simulink model "TENSGwithGFM_electromechanical"  (R2020a)
settings: Solver=VariableStepAuto  StartTime=0.0  StopTime=10.0  FixedStep=0.01  RelTol=1e-3
values from neighbouring files (symbols this model uses):
  GFMInit = GFMSimple_init(resultsac,GFM_in_gidx)    [init.m]
  GSGInit =     [SixGFMconfig.mat]    (also in eightGFMconfig.mat; fourGFMconfig.mat; init.m = SG_init(resultsac,SG_in_gidx); tenGFMconfig.mat)
  Pload = [0 0 0 0 0 0 0 0 0 0 0 0 ... (39 elements, 39x1)]    [SixGFMconfig.mat]    (also in eightGFMconfig.mat; fourGFMconfig.mat; init.m = -resultsac.bus{[CZno,CPno],3}/1000; tenGFMconfig.mat)
  Qload = -resultsac.bus{[CZno,CPno],4}/1000    [init.m]
  Satura = Ses_g(GFM_in_gidx)    [init.m]
  U = [1.0278659059 0.919047677638 0.824047236404 0.914672565668 0.984993620745 0.992890253418 1.00337242347 1.00687710353 1.06162588537 0.973548635627 0.980333735458 0.971076509646 ... (88 elements, 88x1)]    [SixGFMconfig.mat]    (also in eightGFMconfig.mat; fourGFMconfig.mat; init.m = resultsac.bus{:,8}.*exp(1i*(resultsac.bus{:,9})/180*pi); tenGFMconfig.mat)
  Vload = Vbus([CZno,CPno])    [init.m]
  W0 = wB    (= 314.159265359)    [init.m]
  Y_new = [-5.55111512313e-17 -2.77555756156e-17 0 0 0 0 0 0 0 0 0 0 ... (7744 elements, 88x88)]    [SixGFMconfig.mat]    (also in eightGFMconfig.mat; fourGFMconfig.mat; init.m = Y_new([CSno,CPno,GFMother],[CSno,CPno,GFMother]); kron.m = Y)
libraries: eeTransforms x45, simulink_extras x10
(part 3 of 3)

== system TENSGwithGFM_electromechanical/SG1_6 ==
  note: $\[\begin{array}{l} \\ \left\{ \begin{array}{l} {{T'}_d}{{\dot E'}_q} = {E_{fd}} - {{E'}_q} - \left( {{X_d} - {{X'}_d}} \right){I_d}\\ {V_d} = {X_q}{I_q}\\ {V_q} = {{E'}_q} - {{X'}_d}{I_d} \end{array} \right. \end{array}\]$ ${{T'}_d}\dot{{{E'}_q}}=E_{fd}-{E'}_q-(X_d-{X'}_d)I_d \[{V_d} = {X_q}{I_q}\] \[{V_q} = {{E'}_q} - {{X'}_d}{I_d}\]$
  note: AVR
  note: 绕组
  Vxy : Inport
  step : Inport  Port=2
  Clarke to Park Angle Transform1 : eeTransforms/Clarke to Park Angle Transform  AxisAlignment=D-axis
      settings: SourceProductBaseCode=PS
  Constant : Constant  Value=Vref0
  Constant1 : Constant  Value=Pref
  Demux2 : Demux  Outputs=3
  Demux3 : Demux  Outputs=3
  Fcn : Fcn  Expr=sqrt(u(1)^2+u(2)^2)
  Fcn1 : Fcn  Expr=u(1)*u(3)+u(2)*u(4)
  Gain : Gain  Gain=1/Xd1
  Gain1 : Gain  Gain=1/(2*pi)
  Gain10 : Gain  Gain=Xd-Xd1
  Gain12 : Gain  Gain=1/Xq
  Gain13 : Gain  Gain=1/JSG
  Gain14 : Gain  Gain=DSG
  Gain15 : Gain  Gain=W0
  I1 : Constant  Value=0
  I3 : Constant  Value=0
  Integrator1 : Integrator  InitialCondition=theta0
  Integrator5 : Integrator
  Mux{,3..5,7} (5 alike) : Mux  Inputs=2
  Mux1 : Mux
  Park to Clarke Angle Transform2 : eeTransforms/Park to Clarke Angle Transform  AxisAlignment=D-axis
      settings: SourceProductBaseCode=PS
  R_choke15 : Gain  Gain=1/Td1  SaturateOnIntegerOverflow=on  OutDataTypeStr=Inherit: Same as input  ParamDataTypeStr=Inherit: Same as input
  Scope{,1..6,8} (8 alike) : Scope
  Sum : Sum  Inputs=|++
  Sum14 : Sum  Inputs=+--  SaturateOnIntegerOverflow=on
  Sum15 : Sum  Inputs=+-  SaturateOnIntegerOverflow=on
  Sum16 : Sum  Inputs=+---
  Sum18 : Sum  Inputs=|+-
  Terminator2 : Terminator
  Terminator3 : Terminator
  Transfer Fcn (with initial outputs) : simulink_extras/Additional Linear/Transfer Fcn (with initial outputs)  N=[KAVR]  D=[TAVR 1]  Y0=Efd0  U0=0
  U1xy1 : Integrator  InitialCondition=Eq10
  govern system : Subsystem
  Ixy : Outport
  f : Outport  Port=2
  P : Outport  Port=3
  wires:
  Integrator1/1 -> [thetasg], Scope1/1
  Gain15/1 -> Gain1/1, Integrator1/1
  [Efd] -> Sum14/1
  Sum14/1 -> R_choke15/1
  R_choke15/1 -> U1xy1/1
  U1xy1/1 -> Scope6/1, [Eq1], Sum14/2
  [Id] -> Gain10/1
  Gain10/1 -> Sum14/3
  [Eq1] -> Scope3/1, Sum15/1
  [Vq] -> Sum15/2
  Sum15/1 -> Gain/1
  [Vd] -> Gain12/1
  Gain12/1 -> [Iq]
  govern system/1(PM) -> Sum16/3
  Gain13/1 -> Integrator5/1
  Gain14/1 -> Sum16/4
  Sum16/1 -> Gain13/1
  Integrator5/1 -> Gain15/1, govern system/1(deltaw), Gain14/1  "p.u."
  Fcn1/1 -> P/1, Scope5/1, Sum16/2
  Sum18/1 -> Transfer Fcn (with initial outputs)/1, Scope2/1
  [Vd] -> Mux/1
  [Vq] -> Mux/2
  Mux/1 -> Fcn/1
  Constant/1 -> Sum18/1
  Transfer Fcn (with initial outputs)/1 -> Scope8/1, [Efd]
  [Vq] -> Mux1/2
  [Vd] -> Mux1/1
  [Id] -> Mux1/3
  [Iq] -> Mux1/4
  Mux1/1 -> Fcn1/1
  [Iq] -> Mux3/2
  [Id] -> Mux3/1
  Mux4/1 -> Park to Clarke Angle Transform2/1
  I1/1 -> Mux4/2
  Mux3/1 -> Mux4/1
  Demux2/3 -> Terminator2/1
  Demux2/2 -> Mux5/2
  Mux5/1 -> [Ixy], Scope4/1
  [thetasg] -> Park to Clarke Angle Transform2/2
  Park to Clarke Angle Transform2/1 -> Demux2/1  "Vxy"
  Demux2/1 -> Mux5/1
  Vxy/1 -> [Vxy]
  [Ixy] -> Ixy/1
  Fcn/1 -> Scope/1, Sum18/2
  Mux7/1 -> Clarke to Park Angle Transform1/1
  Clarke to Park Angle Transform1/1 -> Demux3/1
  [Vxy] -> Mux7/1
  [thetasg] -> Clarke to Park Angle Transform1/2
  I3/1 -> Mux7/2
  Demux3/3 -> Terminator3/1
  Demux3/2 -> [Vq]
  Demux3/1 -> [Vd]
  Gain/1 -> [Id]
  Gain1/1 -> f/1
  Constant1/1 -> Sum/2
  Sum/1 -> Sum16/1
  step/1 -> Sum/1

== system TENSGwithGFM_electromechanical/SG1_7 ==
  note: $\[\begin{array}{l} \\ \left\{ \begin{array}{l} {{T'}_d}{{\dot E'}_q} = {E_{fd}} - {{E'}_q} - \left( {{X_d} - {{X'}_d}} \right){I_d}\\ {V_d} = {X_q}{I_q}\\ {V_q} = {{E'}_q} - {{X'}_d}{I_d} \end{array} \right. \end{array}\]$ ${{T'}_d}\dot{{{E'}_q}}=E_{fd}-{E'}_q-(X_d-{X'}_d)I_d \[{V_d} = {X_q}{I_q}\] \[{V_q} = {{E'}_q} - {{X'}_d}{I_d}\]$
  note: AVR
  note: 绕组
  Vxy : Inport
  step : Inport  Port=2
  Clarke to Park Angle Transform1 : eeTransforms/Clarke to Park Angle Transform  AxisAlignment=D-axis
      settings: SourceProductBaseCode=PS
  Constant : Constant  Value=Vref0
  Constant1 : Constant  Value=Pref
  Demux2 : Demux  Outputs=3
  Demux3 : Demux  Outputs=3
  Fcn : Fcn  Expr=sqrt(u(1)^2+u(2)^2)
  Fcn1 : Fcn  Expr=u(1)*u(3)+u(2)*u(4)
  Gain : Gain  Gain=1/Xd1
  Gain1 : Gain  Gain=1/(2*pi)
  Gain10 : Gain  Gain=Xd-Xd1
  Gain12 : Gain  Gain=1/Xq
  Gain13 : Gain  Gain=1/JSG
  Gain14 : Gain  Gain=DSG
  Gain15 : Gain  Gain=W0
  I1 : Constant  Value=0
  I3 : Constant  Value=0
  Integrator1 : Integrator  InitialCondition=theta0
  Integrator5 : Integrator
  Mux{,3..5,7} (5 alike) : Mux  Inputs=2
  Mux1 : Mux
  Park to Clarke Angle Transform2 : eeTransforms/Park to Clarke Angle Transform  AxisAlignment=D-axis
      settings: SourceProductBaseCode=PS
  R_choke15 : Gain  Gain=1/Td1  SaturateOnIntegerOverflow=on  OutDataTypeStr=Inherit: Same as input  ParamDataTypeStr=Inherit: Same as input
  Scope{,1..6,8} (8 alike) : Scope
  Sum : Sum  Inputs=|++
  Sum14 : Sum  Inputs=+--  SaturateOnIntegerOverflow=on
  Sum15 : Sum  Inputs=+-  SaturateOnIntegerOverflow=on
  Sum16 : Sum  Inputs=+---
  Sum18 : Sum  Inputs=|+-
  Terminator2 : Terminator
  Terminator3 : Terminator
  Transfer Fcn (with initial outputs) : simulink_extras/Additional Linear/Transfer Fcn (with initial outputs)  N=[KAVR]  D=[TAVR 1]  Y0=Efd0  U0=0
  U1xy1 : Integrator  InitialCondition=Eq10
  govern system : Subsystem
  Ixy : Outport
  f : Outport  Port=2
  P : Outport  Port=3
  wires:
  Integrator1/1 -> [thetasg], Scope1/1
  Gain15/1 -> Gain1/1, Integrator1/1
  [Efd] -> Sum14/1
  Sum14/1 -> R_choke15/1
  R_choke15/1 -> U1xy1/1
  U1xy1/1 -> Scope6/1, [Eq1], Sum14/2
  [Id] -> Gain10/1
  Gain10/1 -> Sum14/3
  [Eq1] -> Scope3/1, Sum15/1
  [Vq] -> Sum15/2
  Sum15/1 -> Gain/1
  [Vd] -> Gain12/1
  Gain12/1 -> [Iq]
  govern system/1(PM) -> Sum16/3
  Gain13/1 -> Integrator5/1
  Gain14/1 -> Sum16/4
  Sum16/1 -> Gain13/1
  Integrator5/1 -> Gain15/1, govern system/1(deltaw), Gain14/1  "p.u."
  Fcn1/1 -> P/1, Scope5/1, Sum16/2
  Sum18/1 -> Transfer Fcn (with initial outputs)/1, Scope2/1
  [Vd] -> Mux/1
  [Vq] -> Mux/2
  Mux/1 -> Fcn/1
  Constant/1 -> Sum18/1
  Transfer Fcn (with initial outputs)/1 -> Scope8/1, [Efd]
  [Vq] -> Mux1/2
  [Vd] -> Mux1/1
  [Id] -> Mux1/3
  [Iq] -> Mux1/4
  Mux1/1 -> Fcn1/1
  [Iq] -> Mux3/2
  [Id] -> Mux3/1
  Mux4/1 -> Park to Clarke Angle Transform2/1
  I1/1 -> Mux4/2
  Mux3/1 -> Mux4/1
  Demux2/3 -> Terminator2/1
  Demux2/2 -> Mux5/2
  Mux5/1 -> [Ixy], Scope4/1
  [thetasg] -> Park to Clarke Angle Transform2/2
  Park to Clarke Angle Transform2/1 -> Demux2/1  "Vxy"
  Demux2/1 -> Mux5/1
  Vxy/1 -> [Vxy]
  [Ixy] -> Ixy/1
  Fcn/1 -> Scope/1, Sum18/2
  Mux7/1 -> Clarke to Park Angle Transform1/1
  Clarke to Park Angle Transform1/1 -> Demux3/1
  [Vxy] -> Mux7/1
  [thetasg] -> Clarke to Park Angle Transform1/2
  I3/1 -> Mux7/2
  Demux3/3 -> Terminator3/1
  Demux3/2 -> [Vq]
  Demux3/1 -> [Vd]
  Gain/1 -> [Id]
  Gain1/1 -> f/1
  Constant1/1 -> Sum/2
  Sum/1 -> Sum16/1
  step/1 -> Sum/1

== system TENSGwithGFM_electromechanical/SG1_8 ==
  note: $\[\begin{array}{l} \\ \left\{ \begin{array}{l} {{T'}_d}{{\dot E'}_q} = {E_{fd}} - {{E'}_q} - \left( {{X_d} - {{X'}_d}} \right){I_d}\\ {V_d} = {X_q}{I_q}\\ {V_q} = {{E'}_q} - {{X'}_d}{I_d} \end{array} \right. \end{array}\]$ ${{T'}_d}\dot{{{E'}_q}}=E_{fd}-{E'}_q-(X_d-{X'}_d)I_d \[{V_d} = {X_q}{I_q}\] \[{V_q} = {{E'}_q} - {{X'}_d}{I_d}\]$
  note: AVR
  note: 绕组
  Vxy : Inport
  step : Inport  Port=2
  Clarke to Park Angle Transform1 : eeTransforms/Clarke to Park Angle Transform  AxisAlignment=D-axis
      settings: SourceProductBaseCode=PS
  Constant : Constant  Value=Vref0
  Constant1 : Constant  Value=Pref
  Demux2 : Demux  Outputs=3
  Demux3 : Demux  Outputs=3
  Fcn : Fcn  Expr=sqrt(u(1)^2+u(2)^2)
  Fcn1 : Fcn  Expr=u(1)*u(3)+u(2)*u(4)
  Gain : Gain  Gain=1/Xd1
  Gain1 : Gain  Gain=1/(2*pi)
  Gain10 : Gain  Gain=Xd-Xd1
  Gain12 : Gain  Gain=1/Xq
  Gain13 : Gain  Gain=1/JSG
  Gain14 : Gain  Gain=DSG
  Gain15 : Gain  Gain=W0
  I1 : Constant  Value=0
  I3 : Constant  Value=0
  Integrator1 : Integrator  InitialCondition=theta0
  Integrator5 : Integrator
  Mux{,3..5,7} (5 alike) : Mux  Inputs=2
  Mux1 : Mux
  Park to Clarke Angle Transform2 : eeTransforms/Park to Clarke Angle Transform  AxisAlignment=D-axis
      settings: SourceProductBaseCode=PS
  R_choke15 : Gain  Gain=1/Td1  SaturateOnIntegerOverflow=on  OutDataTypeStr=Inherit: Same as input  ParamDataTypeStr=Inherit: Same as input
  Scope{,1..6,8} (8 alike) : Scope
  Sum : Sum  Inputs=|++
  Sum14 : Sum  Inputs=+--  SaturateOnIntegerOverflow=on
  Sum15 : Sum  Inputs=+-  SaturateOnIntegerOverflow=on
  Sum16 : Sum  Inputs=+---
  Sum18 : Sum  Inputs=|+-
  Terminator2 : Terminator
  Terminator3 : Terminator
  Transfer Fcn (with initial outputs) : simulink_extras/Additional Linear/Transfer Fcn (with initial outputs)  N=[KAVR]  D=[TAVR 1]  Y0=Efd0  U0=0
  U1xy1 : Integrator  InitialCondition=Eq10
  govern system : Subsystem
  Ixy : Outport
  f : Outport  Port=2
  P : Outport  Port=3
  wires:
  Integrator1/1 -> [thetasg], Scope1/1
  Gain15/1 -> Gain1/1, Integrator1/1
  [Efd] -> Sum14/1
  Sum14/1 -> R_choke15/1
  R_choke15/1 -> U1xy1/1
  U1xy1/1 -> Scope6/1, [Eq1], Sum14/2
  [Id] -> Gain10/1
  Gain10/1 -> Sum14/3
  [Eq1] -> Scope3/1, Sum15/1
  [Vq] -> Sum15/2
  Sum15/1 -> Gain/1
  [Vd] -> Gain12/1
  Gain12/1 -> [Iq]
  govern system/1(PM) -> Sum16/3
  Gain13/1 -> Integrator5/1
  Gain14/1 -> Sum16/4
  Sum16/1 -> Gain13/1
  Integrator5/1 -> Gain15/1, govern system/1(deltaw), Gain14/1  "p.u."
  Fcn1/1 -> P/1, Scope5/1, Sum16/2
  Sum18/1 -> Transfer Fcn (with initial outputs)/1, Scope2/1
  [Vd] -> Mux/1
  [Vq] -> Mux/2
  Mux/1 -> Fcn/1
  Constant/1 -> Sum18/1
  Transfer Fcn (with initial outputs)/1 -> Scope8/1, [Efd]
  [Vq] -> Mux1/2
  [Vd] -> Mux1/1
  [Id] -> Mux1/3
  [Iq] -> Mux1/4
  Mux1/1 -> Fcn1/1
  [Iq] -> Mux3/2
  [Id] -> Mux3/1
  Mux4/1 -> Park to Clarke Angle Transform2/1
  I1/1 -> Mux4/2
  Mux3/1 -> Mux4/1
  Demux2/3 -> Terminator2/1
  Demux2/2 -> Mux5/2
  Mux5/1 -> [Ixy], Scope4/1
  [thetasg] -> Park to Clarke Angle Transform2/2
  Park to Clarke Angle Transform2/1 -> Demux2/1  "Vxy"
  Demux2/1 -> Mux5/1
  Vxy/1 -> [Vxy]
  [Ixy] -> Ixy/1
  Fcn/1 -> Scope/1, Sum18/2
  Mux7/1 -> Clarke to Park Angle Transform1/1
  Clarke to Park Angle Transform1/1 -> Demux3/1
  [Vxy] -> Mux7/1
  [thetasg] -> Clarke to Park Angle Transform1/2
  I3/1 -> Mux7/2
  Demux3/3 -> Terminator3/1
  Demux3/2 -> [Vq]
  Demux3/1 -> [Vd]
  Gain/1 -> [Id]
  Gain1/1 -> f/1
  Constant1/1 -> Sum/2
  Sum/1 -> Sum16/1
  step/1 -> Sum/1

== system TENSGwithGFM_electromechanical/SG1_9 ==
  note: $\[\begin{array}{l} \\ \left\{ \begin{array}{l} {{T'}_d}{{\dot E'}_q} = {E_{fd}} - {{E'}_q} - \left( {{X_d} - {{X'}_d}} \right){I_d}\\ {V_d} = {X_q}{I_q}\\ {V_q} = {{E'}_q} - {{X'}_d}{I_d} \end{array} \right. \end{array}\]$ ${{T'}_d}\dot{{{E'}_q}}=E_{fd}-{E'}_q-(X_d-{X'}_d)I_d \[{V_d} = {X_q}{I_q}\] \[{V_q} = {{E'}_q} - {{X'}_d}{I_d}\]$
  note: AVR
  note: 绕组
  Vxy : Inport
  step : Inport  Port=2
  Clarke to Park Angle Transform1 : eeTransforms/Clarke to Park Angle Transform  AxisAlignment=D-axis
      settings: SourceProductBaseCode=PS
  Constant : Constant  Value=Vref0
  Constant1 : Constant  Value=Pref
  Demux2 : Demux  Outputs=3
  Demux3 : Demux  Outputs=3
  Fcn : Fcn  Expr=sqrt(u(1)^2+u(2)^2)
  Fcn1 : Fcn  Expr=u(1)*u(3)+u(2)*u(4)
  Gain : Gain  Gain=1/Xd1
  Gain1 : Gain  Gain=1/(2*pi)
  Gain10 : Gain  Gain=Xd-Xd1
  Gain12 : Gain  Gain=1/Xq
  Gain13 : Gain  Gain=1/JSG
  Gain14 : Gain  Gain=DSG
  Gain15 : Gain  Gain=W0
  I1 : Constant  Value=0
  I3 : Constant  Value=0
  Integrator1 : Integrator  InitialCondition=theta0
  Integrator5 : Integrator
  Mux{,3..5,7} (5 alike) : Mux  Inputs=2
  Mux1 : Mux
  Park to Clarke Angle Transform2 : eeTransforms/Park to Clarke Angle Transform  AxisAlignment=D-axis
      settings: SourceProductBaseCode=PS
  R_choke15 : Gain  Gain=1/Td1  SaturateOnIntegerOverflow=on  OutDataTypeStr=Inherit: Same as input  ParamDataTypeStr=Inherit: Same as input
  Scope{,1..6,8} (8 alike) : Scope
  Sum : Sum  Inputs=|++
  Sum14 : Sum  Inputs=+--  SaturateOnIntegerOverflow=on
  Sum15 : Sum  Inputs=+-  SaturateOnIntegerOverflow=on
  Sum16 : Sum  Inputs=+---
  Sum18 : Sum  Inputs=|+-
  Terminator2 : Terminator
  Terminator3 : Terminator
  Transfer Fcn (with initial outputs) : simulink_extras/Additional Linear/Transfer Fcn (with initial outputs)  N=[KAVR]  D=[TAVR 1]  Y0=Efd0  U0=0
  U1xy1 : Integrator  InitialCondition=Eq10
  govern system : Subsystem
  Ixy : Outport
  f : Outport  Port=2
  P : Outport  Port=3
  wires:
  Integrator1/1 -> [thetasg], Scope1/1
  Gain15/1 -> Gain1/1, Integrator1/1
  [Efd] -> Sum14/1
  Sum14/1 -> R_choke15/1
  R_choke15/1 -> U1xy1/1
  U1xy1/1 -> Scope6/1, [Eq1], Sum14/2
  [Id] -> Gain10/1
  Gain10/1 -> Sum14/3
  [Eq1] -> Scope3/1, Sum15/1
  [Vq] -> Sum15/2
  Sum15/1 -> Gain/1
  [Vd] -> Gain12/1
  Gain12/1 -> [Iq]
  govern system/1(PM) -> Sum16/3
  Gain13/1 -> Integrator5/1
  Gain14/1 -> Sum16/4
  Sum16/1 -> Gain13/1
  Integrator5/1 -> Gain15/1, govern system/1(deltaw), Gain14/1  "p.u."
  Fcn1/1 -> P/1, Scope5/1, Sum16/2
  Sum18/1 -> Transfer Fcn (with initial outputs)/1, Scope2/1
  [Vd] -> Mux/1
  [Vq] -> Mux/2
  Mux/1 -> Fcn/1
  Constant/1 -> Sum18/1
  Transfer Fcn (with initial outputs)/1 -> Scope8/1, [Efd]
  [Vq] -> Mux1/2
  [Vd] -> Mux1/1
  [Id] -> Mux1/3
  [Iq] -> Mux1/4
  Mux1/1 -> Fcn1/1
  [Iq] -> Mux3/2
  [Id] -> Mux3/1
  Mux4/1 -> Park to Clarke Angle Transform2/1
  I1/1 -> Mux4/2
  Mux3/1 -> Mux4/1
  Demux2/3 -> Terminator2/1
  Demux2/2 -> Mux5/2
  Mux5/1 -> [Ixy], Scope4/1
  [thetasg] -> Park to Clarke Angle Transform2/2
  Park to Clarke Angle Transform2/1 -> Demux2/1  "Vxy"
  Demux2/1 -> Mux5/1
  Vxy/1 -> [Vxy]
  [Ixy] -> Ixy/1
  Fcn/1 -> Scope/1, Sum18/2
  Mux7/1 -> Clarke to Park Angle Transform1/1
  Clarke to Park Angle Transform1/1 -> Demux3/1
  [Vxy] -> Mux7/1
  [thetasg] -> Clarke to Park Angle Transform1/2
  I3/1 -> Mux7/2
  Demux3/3 -> Terminator3/1
  Demux3/2 -> [Vq]
  Demux3/1 -> [Vd]
  Gain/1 -> [Id]
  Gain1/1 -> f/1
  Constant1/1 -> Sum/2
  Sum/1 -> Sum16/1
  step/1 -> Sum/1

== system TENSGwithGFM_electromechanical/Simple GFL ==
  Vxy : Inport
  Clarke to Park Angle Transform1 : eeTransforms/Clarke to Park Angle Transform  AxisAlignment=D-axis
      settings: SourceProductBaseCode=PS
  Constant1 : Constant  Value=0
  Demux : Demux  Outputs=3
  Demux1 : Demux  Outputs=3
  Fcn : Fcn  Expr=(u(3)*u(1)+u(2)*u(4))/(u(3)^2+u(4)^2)
  Fcn1 : Fcn  Expr=(-u(3)*u(2)+u(1)*u(4))/(u(3)^2+u(4)^2)
  Gain1 : Gain  Gain=1/TO
  Gain2 : Gain  Gain=1/TO
  Gain3 : Gain  Gain=KP
  Gain4 : Gain  Gain=KI
  Gain5 : Gain  Gain=1/TF
  Gain6 : Gain  Gain=W0
  Gain7 : Gain  Gain=JGFL
  Gain8 : Gain  Gain=DGFL
  Gain9 : Gain  Gain=1/TD
  Integrator1 : Integrator  InitialCondition=Id0
  Integrator2 : Integrator
  Integrator3 : Integrator
  Integrator4 : Integrator  InitialCondition=theta
  Integrator5 : Integrator  InitialCondition=Iq0
  Integrator6 : Integrator  InitialCondition=Pref
  Mux : Mux
  Mux1 : Mux  Inputs=3
  Mux2 : Mux  Inputs=2
  Mux3 : Mux  Inputs=2
  Park to Clarke Angle Transform2 : eeTransforms/Park to Clarke Angle Transform  AxisAlignment=D-axis
      settings: SourceProductBaseCode=PS
  Pref1 : Constant  Value=Pref
  Product2 : Product
  Qref1 : Constant  Value=0
  Qref2 : Constant  Value=Qref
  Scope2 : Scope
  Scope3 : Scope
  Scope5 : Scope
  Sum of Elements : Sum  Inputs=+
  Sum{1..2,4,7} (4 alike) : Sum  Inputs=|+-
  Sum3 : Sum  Inputs=|++
  Sum6 : Sum  Inputs=-+-
  Terminator : Terminator
  Terminator1 : Terminator
  Ixy : Outport
  PES : Outport  Port=2
  wires:
  Gain6/1 -> Integrator4/1
  Clarke to Park Angle Transform1/1 -> Demux1/1
  Fcn1/1 -> Sum2/1
  Integrator2/1 -> Sum3/2
  [Vq] -> Mux/4
  Sum4/1 -> Gain5/1
  Gain5/1 -> [dwplldt], Integrator3/1
  Sum3/1 -> Sum4/1
  [Vq] -> Scope3/1, Gain4/1, Gain3/1
  Fcn/1 -> Sum1/1
  Gain4/1 -> Integrator2/1
  Demux1/1 -> [Vd]
  Gain7/1 -> Sum6/1
  Demux1/2 -> [Vq]
  Mux/1 -> Fcn1/1, Fcn/1
  Integrator6/1 -> Sum7/2, Mux/1
  Integrator5/1 -> Sum2/2, Mux1/2
  Demux1/3 -> Terminator/1
  Integrator4/1 -> Park to Clarke Angle Transform2/2, Clarke to Park Angle Transform1/2  "theta"
  Mux1/1 -> Scope5/1, Park to Clarke Angle Transform2/1
  [Vd] -> Mux/3
  Integrator3/1 -> Gain6/1, Sum4/2, Scope2/1, [wpll]
  Gain3/1 -> Sum3/1
  Gain8/1 -> Sum6/3
  Integrator1/1 -> Mux1/1, Sum1/2
  [wpll] -> Gain8/1
  [dwplldt] -> Gain7/1
  Qref1/1 -> Mux1/3
  Qref2/1 -> Mux/2
  Gain1/1 -> Integrator1/1
  Sum1/1 -> Gain1/1
  Sum2/1 -> Gain2/1
  Gain2/1 -> Integrator5/1
  Sum6/1 -> Sum7/1
  Sum7/1 -> Gain9/1
  Gain9/1 -> Integrator6/1
  Mux2/1 -> Clarke to Park Angle Transform1/1
  Vxy/1 -> Product2/1, Mux2/1
  Constant1/1 -> Mux2/2
  Park to Clarke Angle Transform2/1 -> Demux/1  "Ixy"
  Demux/3 -> Terminator1/1
  Demux/1 -> Mux3/1
  Demux/2 -> Mux3/2
  Mux3/1 -> Product2/2, Ixy/1
  Pref1/1 -> Sum6/2
  Product2/1 -> Sum of Elements/1
  Sum of Elements/1 -> PES/1

== system TENSGwithGFM_electromechanical/Simple GFL1 ==
  Vxy : Inport
  Clarke to Park Angle Transform1 : eeTransforms/Clarke to Park Angle Transform  AxisAlignment=D-axis
      settings: SourceProductBaseCode=PS
  Constant1 : Constant  Value=0
  Demux : Demux  Outputs=3
  Demux1 : Demux  Outputs=3
  Fcn : Fcn  Expr=(u(3)*u(1)+u(2)*u(4))/(u(3)^2+u(4)^2)
  Fcn1 : Fcn  Expr=(-u(3)*u(2)+u(1)*u(4))/(u(3)^2+u(4)^2)
  Gain1 : Gain  Gain=1/TO
  Gain2 : Gain  Gain=1/TO
  Gain3 : Gain  Gain=KP
  Gain4 : Gain  Gain=KI
  Gain5 : Gain  Gain=1/TF
  Gain6 : Gain  Gain=W0
  Gain7 : Gain  Gain=JGFL
  Gain8 : Gain  Gain=DGFL
  Gain9 : Gain  Gain=1/TD
  Integrator1 : Integrator  InitialCondition=Id0
  Integrator2 : Integrator
  Integrator3 : Integrator
  Integrator4 : Integrator  InitialCondition=theta
  Integrator5 : Integrator  InitialCondition=Iq0
  Integrator6 : Integrator  InitialCondition=Pref
  Mux : Mux
  Mux1 : Mux  Inputs=3
  Mux2 : Mux  Inputs=2
  Mux3 : Mux  Inputs=2
  Park to Clarke Angle Transform2 : eeTransforms/Park to Clarke Angle Transform  AxisAlignment=D-axis
      settings: SourceProductBaseCode=PS
  Pref1 : Constant  Value=Pref
  Product2 : Product
  Qref1 : Constant  Value=0
  Qref2 : Constant  Value=Qref
  Scope2 : Scope
  Scope3 : Scope
  Scope5 : Scope
  Sum of Elements : Sum  Inputs=+
  Sum{1..2,4,7} (4 alike) : Sum  Inputs=|+-
  Sum3 : Sum  Inputs=|++
  Sum6 : Sum  Inputs=-+-
  Terminator : Terminator
  Terminator1 : Terminator
  Ixy : Outport
  PES : Outport  Port=2
  wires:
  Gain6/1 -> Integrator4/1
  Clarke to Park Angle Transform1/1 -> Demux1/1
  Fcn1/1 -> Sum2/1
  Integrator2/1 -> Sum3/2
  [Vq] -> Mux/4
  Sum4/1 -> Gain5/1
  Gain5/1 -> [dwplldt], Integrator3/1
  Sum3/1 -> Sum4/1
  [Vq] -> Scope3/1, Gain4/1, Gain3/1
  Fcn/1 -> Sum1/1
  Gain4/1 -> Integrator2/1
  Demux1/1 -> [Vd]
  Gain7/1 -> Sum6/1
  Demux1/2 -> [Vq]
  Mux/1 -> Fcn1/1, Fcn/1
  Integrator6/1 -> Sum7/2, Mux/1
  Integrator5/1 -> Sum2/2, Mux1/2
  Demux1/3 -> Terminator/1
  Integrator4/1 -> Park to Clarke Angle Transform2/2, Clarke to Park Angle Transform1/2  "theta"
  Mux1/1 -> Scope5/1, Park to Clarke Angle Transform2/1
  [Vd] -> Mux/3
  Integrator3/1 -> Gain6/1, Sum4/2, Scope2/1, [wpll]
  Gain3/1 -> Sum3/1
  Gain8/1 -> Sum6/3
  Integrator1/1 -> Mux1/1, Sum1/2
  [wpll] -> Gain8/1
  [dwplldt] -> Gain7/1
  Qref1/1 -> Mux1/3
  Qref2/1 -> Mux/2
  Gain1/1 -> Integrator1/1
  Sum1/1 -> Gain1/1
  Sum2/1 -> Gain2/1
  Gain2/1 -> Integrator5/1
  Sum6/1 -> Sum7/1
  Sum7/1 -> Gain9/1
  Gain9/1 -> Integrator6/1
  Mux2/1 -> Clarke to Park Angle Transform1/1
  Vxy/1 -> Product2/1, Mux2/1
  Constant1/1 -> Mux2/2
  Park to Clarke Angle Transform2/1 -> Demux/1  "Ixy"
  Demux/3 -> Terminator1/1
  Demux/1 -> Mux3/1
  Demux/2 -> Mux3/2
  Mux3/1 -> Product2/2, Ixy/1
  Pref1/1 -> Sum6/2
  Sum of Elements/1 -> PES/1
  Product2/1 -> Sum of Elements/1

== system TENSGwithGFM_electromechanical/SG1_1/govern system ==
  deltaw : Inport
  Gain2 : Gain  Gain=K1
  Gain3 : Gain  Gain=K3
  Gain4 : Gain  Gain=K5
  Gain5 : Gain  Gain=K7
  Sum1 : Sum  Inputs=|++
  Sum2 : Sum  Inputs=|++
  Sum3 : Sum  Inputs=|++
  Transfer Fcn : TransferFcn  Numerator=[T2 1]  Denominator=[T3 1]
  Transfer Fcn1 : TransferFcn  Numerator=[Ksg]  Denominator=[T1 1]
  Transfer Fcn2 : TransferFcn  Denominator=[T4 1]
  Transfer Fcn3 : TransferFcn  Denominator=[T5 1]
  Transfer Fcn4 : TransferFcn  Denominator=[T6 1]
  Transfer Fcn5 : TransferFcn  Denominator=[T7 1]
  PM : Outport
  wires:
  Sum2/1 -> Sum3/1
  Transfer Fcn3/1 -> Gain3/1, Transfer Fcn4/1
  Transfer Fcn4/1 -> Gain4/1, Transfer Fcn5/1
  Transfer Fcn5/1 -> Gain5/1
  Sum1/1 -> Sum2/1
  Transfer Fcn2/1 -> Gain2/1, Transfer Fcn3/1
  Gain2/1 -> Sum1/1
  Transfer Fcn1/1 -> Transfer Fcn/1
  Gain5/1 -> Sum3/2
  Transfer Fcn/1 -> Transfer Fcn2/1
  deltaw/1 -> Transfer Fcn1/1
  Gain3/1 -> Sum1/2
  Gain4/1 -> Sum2/2
  Sum3/1 -> PM/1

== system TENSGwithGFM_electromechanical/SG1_10/govern system ==
  deltaw : Inport
  Gain2 : Gain  Gain=K1
  Gain3 : Gain  Gain=K3
  Gain4 : Gain  Gain=K5
  Gain5 : Gain  Gain=K7
  Sum1 : Sum  Inputs=|++
  Sum2 : Sum  Inputs=|++
  Sum3 : Sum  Inputs=|++
  Transfer Fcn : TransferFcn  Numerator=[T2 1]  Denominator=[T3 1]
  Transfer Fcn1 : TransferFcn  Numerator=[Ksg]  Denominator=[T1 1]
  Transfer Fcn2 : TransferFcn  Denominator=[T4 1]
  Transfer Fcn3 : TransferFcn  Denominator=[T5 1]
  Transfer Fcn4 : TransferFcn  Denominator=[T6 1]
  Transfer Fcn5 : TransferFcn  Denominator=[T7 1]
  PM : Outport
  wires:
  Sum2/1 -> Sum3/1
  Transfer Fcn3/1 -> Gain3/1, Transfer Fcn4/1
  Transfer Fcn4/1 -> Gain4/1, Transfer Fcn5/1
  Transfer Fcn5/1 -> Gain5/1
  Sum1/1 -> Sum2/1
  Transfer Fcn2/1 -> Gain2/1, Transfer Fcn3/1
  Gain2/1 -> Sum1/1
  Transfer Fcn1/1 -> Transfer Fcn/1
  Gain5/1 -> Sum3/2
  Transfer Fcn/1 -> Transfer Fcn2/1
  deltaw/1 -> Transfer Fcn1/1
  Gain3/1 -> Sum1/2
  Gain4/1 -> Sum2/2
  Sum3/1 -> PM/1

== system TENSGwithGFM_electromechanical/SG1_2/govern system ==
  deltaw : Inport
  Gain2 : Gain  Gain=K1
  Gain3 : Gain  Gain=K3
  Gain4 : Gain  Gain=K5
  Gain5 : Gain  Gain=K7
  Sum1 : Sum  Inputs=|++
  Sum2 : Sum  Inputs=|++
  Sum3 : Sum  Inputs=|++
  Transfer Fcn : TransferFcn  Numerator=[T2 1]  Denominator=[T3 1]
  Transfer Fcn1 : TransferFcn  Numerator=[Ksg]  Denominator=[T1 1]
  Transfer Fcn2 : TransferFcn  Denominator=[T4 1]
  Transfer Fcn3 : TransferFcn  Denominator=[T5 1]
  Transfer Fcn4 : TransferFcn  Denominator=[T6 1]
  Transfer Fcn5 : TransferFcn  Denominator=[T7 1]
  PM : Outport
  wires:
  Sum2/1 -> Sum3/1
  Transfer Fcn3/1 -> Gain3/1, Transfer Fcn4/1
  Transfer Fcn4/1 -> Gain4/1, Transfer Fcn5/1
  Transfer Fcn5/1 -> Gain5/1
  Sum1/1 -> Sum2/1
  Transfer Fcn2/1 -> Gain2/1, Transfer Fcn3/1
  Gain2/1 -> Sum1/1
  Transfer Fcn1/1 -> Transfer Fcn/1
  Gain5/1 -> Sum3/2
  Transfer Fcn/1 -> Transfer Fcn2/1
  deltaw/1 -> Transfer Fcn1/1
  Gain3/1 -> Sum1/2
  Gain4/1 -> Sum2/2
  Sum3/1 -> PM/1

== system TENSGwithGFM_electromechanical/SG1_3/govern system ==
  deltaw : Inport
  Gain2 : Gain  Gain=K1
  Gain3 : Gain  Gain=K3
  Gain4 : Gain  Gain=K5
  Gain5 : Gain  Gain=K7
  Sum1 : Sum  Inputs=|++
  Sum2 : Sum  Inputs=|++
  Sum3 : Sum  Inputs=|++
  Transfer Fcn : TransferFcn  Numerator=[T2 1]  Denominator=[T3 1]
  Transfer Fcn1 : TransferFcn  Numerator=[Ksg]  Denominator=[T1 1]
  Transfer Fcn2 : TransferFcn  Denominator=[T4 1]
  Transfer Fcn3 : TransferFcn  Denominator=[T5 1]
  Transfer Fcn4 : TransferFcn  Denominator=[T6 1]
  Transfer Fcn5 : TransferFcn  Denominator=[T7 1]
  PM : Outport
  wires:
  Sum2/1 -> Sum3/1
  Transfer Fcn3/1 -> Gain3/1, Transfer Fcn4/1
  Transfer Fcn4/1 -> Gain4/1, Transfer Fcn5/1
  Transfer Fcn5/1 -> Gain5/1
  Sum1/1 -> Sum2/1
  Transfer Fcn2/1 -> Gain2/1, Transfer Fcn3/1
  Gain2/1 -> Sum1/1
  Transfer Fcn1/1 -> Transfer Fcn/1
  Gain5/1 -> Sum3/2
  Transfer Fcn/1 -> Transfer Fcn2/1
  deltaw/1 -> Transfer Fcn1/1
  Gain3/1 -> Sum1/2
  Gain4/1 -> Sum2/2
  Sum3/1 -> PM/1

== system TENSGwithGFM_electromechanical/SG1_4/govern system ==
  deltaw : Inport
  Gain2 : Gain  Gain=K1
  Gain3 : Gain  Gain=K3
  Gain4 : Gain  Gain=K5
  Gain5 : Gain  Gain=K7
  Sum1 : Sum  Inputs=|++
  Sum2 : Sum  Inputs=|++
  Sum3 : Sum  Inputs=|++
  Transfer Fcn : TransferFcn  Numerator=[T2 1]  Denominator=[T3 1]
  Transfer Fcn1 : TransferFcn  Numerator=[Ksg]  Denominator=[T1 1]
  Transfer Fcn2 : TransferFcn  Denominator=[T4 1]
  Transfer Fcn3 : TransferFcn  Denominator=[T5 1]
  Transfer Fcn4 : TransferFcn  Denominator=[T6 1]
  Transfer Fcn5 : TransferFcn  Denominator=[T7 1]
  PM : Outport
  wires:
  Sum2/1 -> Sum3/1
  Transfer Fcn3/1 -> Gain3/1, Transfer Fcn4/1
  Transfer Fcn4/1 -> Gain4/1, Transfer Fcn5/1
  Transfer Fcn5/1 -> Gain5/1
  Sum1/1 -> Sum2/1
  Transfer Fcn2/1 -> Gain2/1, Transfer Fcn3/1
  Gain2/1 -> Sum1/1
  Transfer Fcn1/1 -> Transfer Fcn/1
  Gain5/1 -> Sum3/2
  Transfer Fcn/1 -> Transfer Fcn2/1
  deltaw/1 -> Transfer Fcn1/1
  Gain3/1 -> Sum1/2
  Gain4/1 -> Sum2/2
  Sum3/1 -> PM/1

== system TENSGwithGFM_electromechanical/SG1_5/govern system ==
  deltaw : Inport
  Gain2 : Gain  Gain=K1
  Gain3 : Gain  Gain=K3
  Gain4 : Gain  Gain=K5
  Gain5 : Gain  Gain=K7
  Sum1 : Sum  Inputs=|++
  Sum2 : Sum  Inputs=|++
  Sum3 : Sum  Inputs=|++
  Transfer Fcn : TransferFcn  Numerator=[T2 1]  Denominator=[T3 1]
  Transfer Fcn1 : TransferFcn  Numerator=[Ksg]  Denominator=[T1 1]
  Transfer Fcn2 : TransferFcn  Denominator=[T4 1]
  Transfer Fcn3 : TransferFcn  Denominator=[T5 1]
  Transfer Fcn4 : TransferFcn  Denominator=[T6 1]
  Transfer Fcn5 : TransferFcn  Denominator=[T7 1]
  PM : Outport
  wires:
  Sum2/1 -> Sum3/1
  Transfer Fcn3/1 -> Gain3/1, Transfer Fcn4/1
  Transfer Fcn4/1 -> Gain4/1, Transfer Fcn5/1
  Transfer Fcn5/1 -> Gain5/1
  Sum1/1 -> Sum2/1
  Transfer Fcn2/1 -> Gain2/1, Transfer Fcn3/1
  Gain2/1 -> Sum1/1
  Transfer Fcn1/1 -> Transfer Fcn/1
  Gain5/1 -> Sum3/2
  Transfer Fcn/1 -> Transfer Fcn2/1
  deltaw/1 -> Transfer Fcn1/1
  Gain3/1 -> Sum1/2
  Gain4/1 -> Sum2/2
  Sum3/1 -> PM/1

== system TENSGwithGFM_electromechanical/SG1_6/govern system ==
  deltaw : Inport
  Gain2 : Gain  Gain=K1
  Gain3 : Gain  Gain=K3
  Gain4 : Gain  Gain=K5
  Gain5 : Gain  Gain=K7
  Sum1 : Sum  Inputs=|++
  Sum2 : Sum  Inputs=|++
  Sum3 : Sum  Inputs=|++
  Transfer Fcn : TransferFcn  Numerator=[T2 1]  Denominator=[T3 1]
  Transfer Fcn1 : TransferFcn  Numerator=[Ksg]  Denominator=[T1 1]
  Transfer Fcn2 : TransferFcn  Denominator=[T4 1]
  Transfer Fcn3 : TransferFcn  Denominator=[T5 1]
  Transfer Fcn4 : TransferFcn  Denominator=[T6 1]
  Transfer Fcn5 : TransferFcn  Denominator=[T7 1]
  PM : Outport
  wires:
  Sum2/1 -> Sum3/1
  Transfer Fcn3/1 -> Gain3/1, Transfer Fcn4/1
  Transfer Fcn4/1 -> Gain4/1, Transfer Fcn5/1
  Transfer Fcn5/1 -> Gain5/1
  Sum1/1 -> Sum2/1
  Transfer Fcn2/1 -> Gain2/1, Transfer Fcn3/1
  Gain2/1 -> Sum1/1
  Transfer Fcn1/1 -> Transfer Fcn/1
  Gain5/1 -> Sum3/2
  Transfer Fcn/1 -> Transfer Fcn2/1
  deltaw/1 -> Transfer Fcn1/1
  Gain3/1 -> Sum1/2
  Gain4/1 -> Sum2/2
  Sum3/1 -> PM/1

== system TENSGwithGFM_electromechanical/SG1_7/govern system ==
  deltaw : Inport
  Gain2 : Gain  Gain=K1
  Gain3 : Gain  Gain=K3
  Gain4 : Gain  Gain=K5
  Gain5 : Gain  Gain=K7
  Sum1 : Sum  Inputs=|++
  Sum2 : Sum  Inputs=|++
  Sum3 : Sum  Inputs=|++
  Transfer Fcn : TransferFcn  Numerator=[T2 1]  Denominator=[T3 1]
  Transfer Fcn1 : TransferFcn  Numerator=[Ksg]  Denominator=[T1 1]
  Transfer Fcn2 : TransferFcn  Denominator=[T4 1]
  Transfer Fcn3 : TransferFcn  Denominator=[T5 1]
  Transfer Fcn4 : TransferFcn  Denominator=[T6 1]
  Transfer Fcn5 : TransferFcn  Denominator=[T7 1]
  PM : Outport
  wires:
  Sum2/1 -> Sum3/1
  Transfer Fcn3/1 -> Gain3/1, Transfer Fcn4/1
  Transfer Fcn4/1 -> Gain4/1, Transfer Fcn5/1
  Transfer Fcn5/1 -> Gain5/1
  Sum1/1 -> Sum2/1
  Transfer Fcn2/1 -> Gain2/1, Transfer Fcn3/1
  Gain2/1 -> Sum1/1
  Transfer Fcn1/1 -> Transfer Fcn/1
  Gain5/1 -> Sum3/2
  Transfer Fcn/1 -> Transfer Fcn2/1
  deltaw/1 -> Transfer Fcn1/1
  Gain3/1 -> Sum1/2
  Gain4/1 -> Sum2/2
  Sum3/1 -> PM/1

== system TENSGwithGFM_electromechanical/SG1_8/govern system ==
  deltaw : Inport
  Gain2 : Gain  Gain=K1
  Gain3 : Gain  Gain=K3
  Gain4 : Gain  Gain=K5
  Gain5 : Gain  Gain=K7
  Sum1 : Sum  Inputs=|++
  Sum2 : Sum  Inputs=|++
  Sum3 : Sum  Inputs=|++
  Transfer Fcn : TransferFcn  Numerator=[T2 1]  Denominator=[T3 1]
  Transfer Fcn1 : TransferFcn  Numerator=[Ksg]  Denominator=[T1 1]
  Transfer Fcn2 : TransferFcn  Denominator=[T4 1]
  Transfer Fcn3 : TransferFcn  Denominator=[T5 1]
  Transfer Fcn4 : TransferFcn  Denominator=[T6 1]
  Transfer Fcn5 : TransferFcn  Denominator=[T7 1]
  PM : Outport
  wires:
  Sum2/1 -> Sum3/1
  Transfer Fcn3/1 -> Gain3/1, Transfer Fcn4/1
  Transfer Fcn4/1 -> Gain4/1, Transfer Fcn5/1
  Transfer Fcn5/1 -> Gain5/1
  Sum1/1 -> Sum2/1
  Transfer Fcn2/1 -> Gain2/1, Transfer Fcn3/1
  Gain2/1 -> Sum1/1
  Transfer Fcn1/1 -> Transfer Fcn/1
  Gain5/1 -> Sum3/2
  Transfer Fcn/1 -> Transfer Fcn2/1
  deltaw/1 -> Transfer Fcn1/1
  Gain3/1 -> Sum1/2
  Gain4/1 -> Sum2/2
  Sum3/1 -> PM/1

== system TENSGwithGFM_electromechanical/SG1_9/govern system ==
  deltaw : Inport
  Gain2 : Gain  Gain=K1
  Gain3 : Gain  Gain=K3
  Gain4 : Gain  Gain=K5
  Gain5 : Gain  Gain=K7
  Sum1 : Sum  Inputs=|++
  Sum2 : Sum  Inputs=|++
  Sum3 : Sum  Inputs=|++
  Transfer Fcn : TransferFcn  Numerator=[T2 1]  Denominator=[T3 1]
  Transfer Fcn1 : TransferFcn  Numerator=[Ksg]  Denominator=[T1 1]
  Transfer Fcn2 : TransferFcn  Denominator=[T4 1]
  Transfer Fcn3 : TransferFcn  Denominator=[T5 1]
  Transfer Fcn4 : TransferFcn  Denominator=[T6 1]
  Transfer Fcn5 : TransferFcn  Denominator=[T7 1]
  PM : Outport
  wires:
  Sum2/1 -> Sum3/1
  Transfer Fcn3/1 -> Gain3/1, Transfer Fcn4/1
  Transfer Fcn4/1 -> Gain4/1, Transfer Fcn5/1
  Transfer Fcn5/1 -> Gain5/1
  Sum1/1 -> Sum2/1
  Transfer Fcn2/1 -> Gain2/1, Transfer Fcn3/1
  Gain2/1 -> Sum1/1
  Transfer Fcn1/1 -> Transfer Fcn/1
  Gain5/1 -> Sum3/2
  Transfer Fcn/1 -> Transfer Fcn2/1
  deltaw/1 -> Transfer Fcn1/1
  Gain3/1 -> Sum1/2
  Gain4/1 -> Sum2/2
  Sum3/1 -> PM/1
